simulink library "simulink_utils"  (Simulink 8.2)
settings: Solver=ode1  StartTime=0.0  StopTime=Inf  FixedStep=0.001  RelTol=1e-3
PostLoadFcn:
  | , if any(exist('dsrtsu_mdlpostloadfcn', 'file') == [2, 3, 6]), try dsrtsu_mdlpostloadfcn('Execute', bdroot); catch fprintf('Error in PostLoadFcn (dsrtsu_mdlpostloadfcn) for model "%s":\n %s\n', bdroot, lasterr); end, end,
libraries: simulink x1
settings Model: DSRTSU_INTERNAL_RTI_VER=450  DSRTSU_INTERNAL_RTI_TYPE=rti1401  Creator=rushk1  LastModifiedBy=rushk1

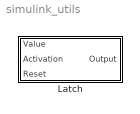
== system simulink_utils ==
  Latch : Subsystem  mask{timestep_threshold=5}
      mask prompts: timestep_threshold "Timestep Threshold:"
      mask DialogControl DescGroupVar Prompt: Timestep Latch
      mask DialogControl DescTextVar Prompt: Latch on a value after a certain number of timesteps have elapsed during which a condition is true.

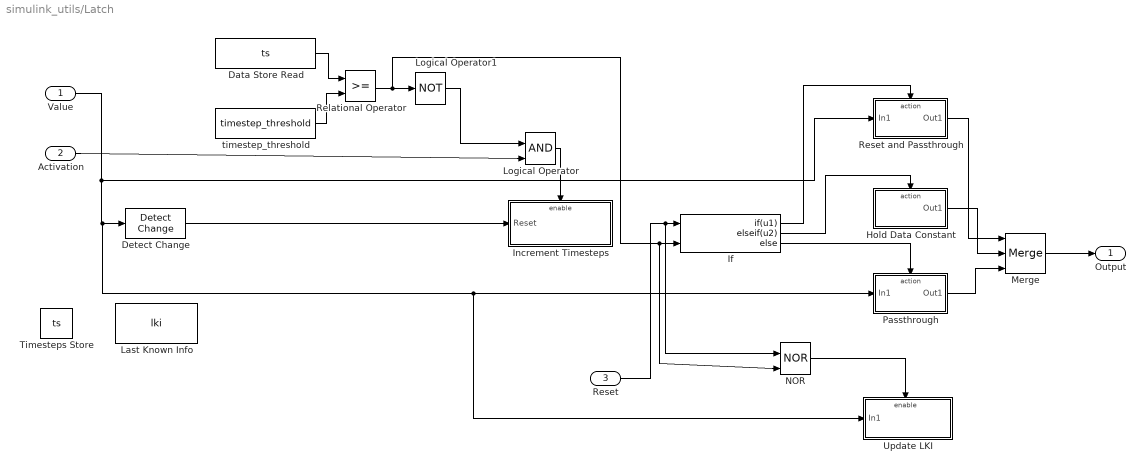
== system simulink_utils/Latch ==
  Value : Inport
  Activation : Inport  Port=2
  Reset : Inport  Port=3
  Data Store Read : DataStoreRead  DataStoreName=ts
  Detect Change : simulink/Logic and Bit Operations/Detect Change  vinit=0  InputProcessing=Inherited  OutDataTypeStr=boolean
  Hold Data Constant : Subsystem  TreatAsAtomicUnit=on
  If : If  NumInputs=2  IfExpression=u1  ElseIfExpressions=u2
  Increment Timesteps : Subsystem  TreatAsAtomicUnit=on
  Last Known Info : DataStoreMemory  DataStoreName=lki  ReadBeforeWriteMsg=warning  WriteAfterWriteMsg=warning  WriteAfterReadMsg=warning
  Logical Operator : Logic  IconShape=distinctive  AllPortsSameDT=off  OutDataTypeStr=boolean
  Logical Operator1 : Logic  Operator=NOT  IconShape=distinctive  AllPortsSameDT=off  OutDataTypeStr=boolean
  Merge : Merge  Inputs=3
  NOR : Logic  Operator=NOR  IconShape=distinctive  AllPortsSameDT=off  OutDataTypeStr=boolean
  Passthrough : Subsystem  TreatAsAtomicUnit=on
  Relational Operator : RelationalOperator  OutDataTypeStr=boolean
  Reset and Passthrough : Subsystem  TreatAsAtomicUnit=on
  Timesteps Store : DataStoreMemory  DataStoreName=ts  ReadBeforeWriteMsg=warning  WriteAfterWriteMsg=warning  WriteAfterReadMsg=warning
  Update LKI : Subsystem  TreatAsAtomicUnit=on
  timestep_threshold : Constant  Value=timestep_threshold
  Output : Outport
  wires:
  Activation/1 -> Logical Operator/2
  Value/1 -> Update LKI/1(In1), Passthrough/1(In1), Detect Change/1, Reset and Passthrough/1(In1)
  Detect Change/1 -> Increment Timesteps/1(Reset)
  If/3 -> Passthrough/Action
  Hold Data Constant/1(Out1) -> Merge/2
  Passthrough/1(Out1) -> Merge/3
  Merge/1 -> Output/1
  timestep_threshold/1 -> Relational Operator/2
  Relational Operator/1 -> NOR/2, If/2, Logical Operator1/1
  Data Store Read/1 -> Relational Operator/1
  Logical Operator1/1 -> Logical Operator/1
  Logical Operator/1 -> Increment Timesteps/Enable
  Reset/1 -> NOR/1, If/1
  If/2 -> Hold Data Constant/Action
  If/1 -> Reset and Passthrough/Action
  Reset and Passthrough/1(Out1) -> Merge/1
  NOR/1 -> Update LKI/Enable

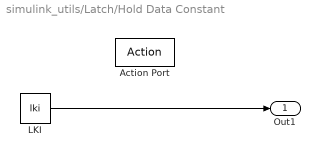
== system simulink_utils/Latch/Hold Data Constant ==
  Action Port : ActionPort  ActionType=elseif
  LKI : DataStoreRead  DataStoreName=lki
  Out1 : Outport
  wires:
  LKI/1 -> Out1/1

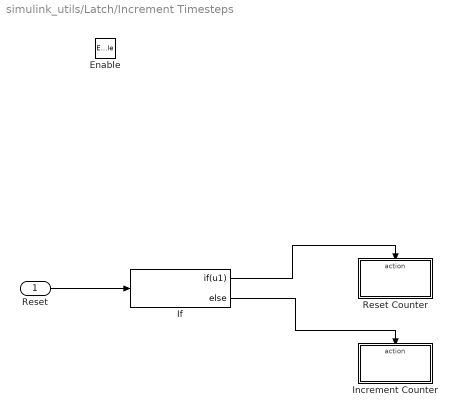
== system simulink_utils/Latch/Increment Timesteps ==
  Reset : Inport
  Enable : EnablePort
  If : If  IfExpression=u1
  Increment Counter : Subsystem  TreatAsAtomicUnit=on
  Reset Counter : Subsystem  TreatAsAtomicUnit=on
  wires:
  Reset/1 -> If/1
  If/1 -> Reset Counter/Action
  If/2 -> Increment Counter/Action

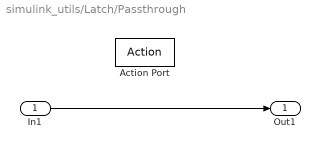
== system simulink_utils/Latch/Passthrough ==
  In1 : Inport
  Action Port : ActionPort  ActionType=else
  Out1 : Outport
  wires:
  In1/1 -> Out1/1

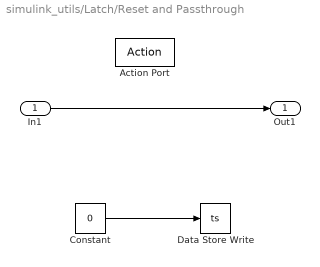
== system simulink_utils/Latch/Reset and Passthrough ==
  In1 : Inport
  Action Port : ActionPort  ActionType=then
  Constant : Constant  Value=0
  Data Store Write : DataStoreWrite  DataStoreName=ts
  Out1 : Outport
  wires:
  In1/1 -> Out1/1
  Constant/1 -> Data Store Write/1

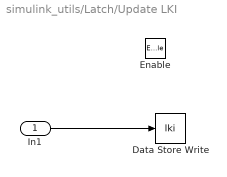
== system simulink_utils/Latch/Update LKI ==
  In1 : Inport
  Enable : EnablePort
  Data Store Write : DataStoreWrite  DataStoreName=lki
  wires:
  In1/1 -> Data Store Write/1

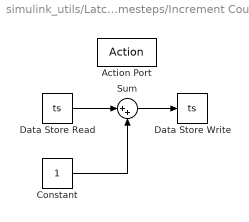
== system simulink_utils/Latch/Increment Timesteps/Increment Counter ==
  Action Port : ActionPort  ActionType=else
  Constant : Constant
  Data Store Read : DataStoreRead  DataStoreName=ts
  Data Store Write : DataStoreWrite  DataStoreName=ts
  Sum : Sum  Inputs=|++
  wires:
  Data Store Read/1 -> Sum/1
  Constant/1 -> Sum/2
  Sum/1 -> Data Store Write/1

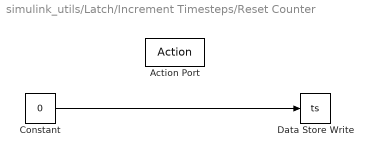
== system simulink_utils/Latch/Increment Timesteps/Reset Counter ==
  Action Port : ActionPort  ActionType=then
  Constant : Constant  Value=0
  Data Store Write : DataStoreWrite  DataStoreName=ts
  wires:
  Constant/1 -> Data Store Write/1
